simulink model "STEVE_ver28"  (R2022a)
settings: Solver=VariableStepAuto  StartTime=0.0  StopTime=Stop_Time  FixedStep=0.000001  RelTol=1e-5
values from neighbouring files (symbols this model uses):
  Bed_ave_OD = (1+Bed_ins_OD)/2    (= 1.667)    [STEVE_initialization.m]    (also in STEVE_running.m = (1+Bed_ins_OD)/2; STEVE_v4_C1Demo_2023_Nominal.m)
  Bed_ins_OD = 2.334    [STEVE_initialization.m]    (also in STEVE_v4_C1Demo_2023_Nominal.m)
  Bed_thickness = 0.049    [STEVE_initialization.m]    (also in STEVE_v4_C1Demo_2023_Nominal.m)
  Belimo_Cv = 16    [STEVE_initialization.m]    (also in STEVE_v4_C1Demo_2023_Nominal.m)
  flow_rate = 8    [STEVE_initialization.m]    (also in STEVE_v4_C1Demo_2023_Nominal.m)
  Heat_ads = 40000    [STEVE_initialization.m]    (also in STEVE_v4_C1Demo_2023_Nominal.m)
  Heater_output = 85.3    [STEVE_initialization.m]    (also in STEVE_v4_C1Demo_2023_Nominal.m)
  L = 0.508    [STEVE_initialization.m]    (also in STEVE_v4_C1Demo_2023_Nominal.m)
  L_inch = L*39.3701    (= 20.0000108)    [STEVE_initialization.m]    (also in STEVE_v4_C1Demo_2023_Nominal.m)
  max_temp = 200+273.15    (= 473.15)    [STEVE_initialization.m]    (also in STEVE_v4_C1Demo_2023_Nominal.m)
  mesh_size = 15    [STEVE_initialization.m]    (also in STEVE_v4_C1Demo_2023_Nominal.m)
  Pipe_ave_HD = (pipe_HD+0.5)/2    (= 0.465)    [STEVE_initialization.m]    (also in STEVE_running.m = (pipe_HD+0.5)/2; STEVE_v4_C1Demo_2023_Nominal.m)
  pipe_HD = 0.43    [STEVE_initialization.m]    (also in STEVE_v4_C1Demo_2023_Nominal.m)
  Ramp_rate = 0.0833    [STEVE_initialization.m]    (also in STEVE_v4_C1Demo_2023_Nominal.m)
  room_pressure = 13.3    [STEVE_initialization.m]    (also in STEVE_v4_C1Demo_2023_Nominal.m)
  t_Total = Adsorption_time + FlowStop_time + Valve_close_Time + Select_valve_close_Time + Pump_down_time + Desorption_time + SelectValve_open_Time + Valve_open_Time    (= 9635)    [STEVE_initialization.m]    (also in STEVE_running.m = Adsorption_time + FlowStop_time + Valve_close_Time + Select_; STEVE_v4_C1Demo_2023_Nominal.m)
libraries: fl_lib x229, nesl_utility x75, slpidlib x2
(part 5 of 5)

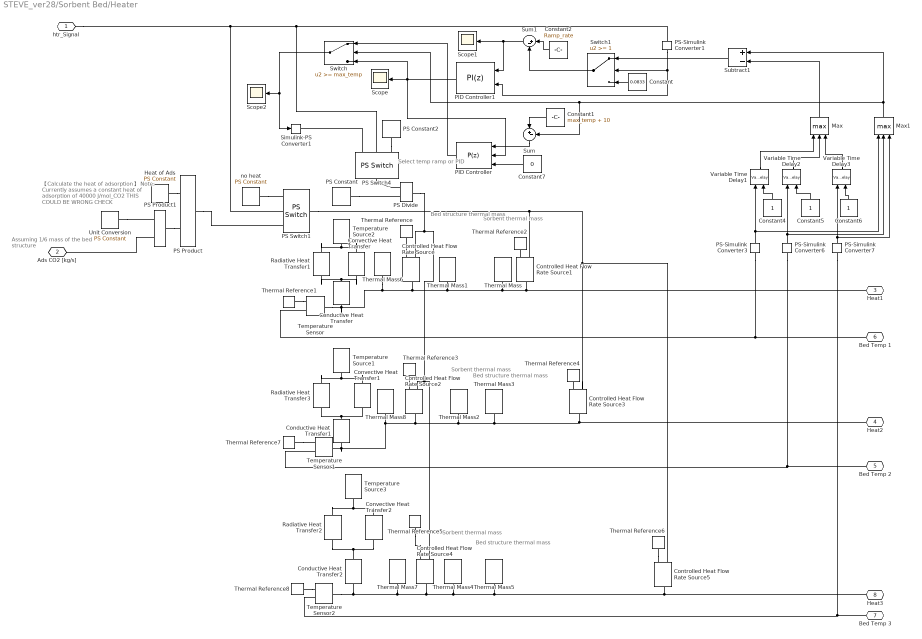
== system STEVE_ver28/Sorbent Bed/Heater ==
  note: 【Calculate the heat of adsorption】
      | Note: Currently assumes a constant heat of adsorption of 40000 J/mol_CO2
      | THIS COULD BE WRONG CHECK
  note: Sorbent thermal mass
  note: Bed structure thermal mass
  note: Bed structure thermal mass
  note: Sorbent thermal mass
  note: Bed structure thermal mass
  note: Sorbent thermal mass
  note: Select temp ramp or PID
  note: Assuming 1/6 mass of the bed structure
  Conductive Heat Transfer : fl_lib/Thermal/Thermal Elements/Conductive Heat Transfer  area=pi*Bed_ave_OD*L_inch/3 in^2  thickness=0.667 in  th_cond=0.07 W/(K*m)  T_specify=off  T_priority=None  T=0 K  T_nominal_specify=off  T_nominal_unit=K  T_nominal_value=1  Q_specify=off  Q_priority=None  Q=0 W  Q_nominal_specify=off  Q_nominal_unit=W  Q_nominal_value=1
      settings: SourceProductBaseCode=PW,SS,VE
  Conductive Heat Transfer1 : fl_lib/Thermal/Thermal Elements/Conductive Heat Transfer  area=pi*Bed_ave_OD*L_inch/3 in^2  thickness=0.667 in  th_cond=0.07 W/(K*m)  T_specify=off  T_priority=None  T=0 K  T_nominal_specify=off  T_nominal_unit=K  T_nominal_value=1  Q_specify=off  Q_priority=None  Q=0 W  Q_nominal_specify=off  Q_nominal_unit=W  Q_nominal_value=1
      settings: SourceProductBaseCode=PW,SS,VE
  Conductive Heat Transfer2 : fl_lib/Thermal/Thermal Elements/Conductive Heat Transfer  area=pi*Bed_ave_OD*L_inch/3 in^2  thickness=0.667 in  th_cond=0.07 W/(K*m)  T_specify=off  T_priority=None  T=0 K  T_nominal_specify=off  T_nominal_unit=K  T_nominal_value=1  Q_specify=off  Q_priority=None  Q=0 W  Q_nominal_specify=off  Q_nominal_unit=W  Q_nominal_value=1
      settings: SourceProductBaseCode=PW,SS,VE
  Constant : Constant  Value=0.0833
  Constant1 : Constant  Value=max_temp + 10
  Constant2 : Constant  Value=Ramp_rate
  Constant4 : Constant
  Constant5 : Constant
  Constant6 : Constant
  Constant7 : Constant  Value=0
  Controlled Heat Flow Rate Source{,1..5} (6 alike) : fl_lib/Thermal/Thermal Sources/Controlled Heat Flow Rate Source
      settings: SourceProductBaseCode=PW,SS,VE
  Convective Heat Transfer : fl_lib/Thermal/Thermal Elements/Convective Heat Transfer  area=pi*Bed_ins_OD*L_inch/3 in^2  heat_tr_coeff=5 W/(K*m^2)  T_specify=off  T_priority=None  T=0 K  T_nominal_specify=off  T_nominal_unit=K  T_nominal_value=1  Q_specify=off  Q_priority=None  Q=0 W  Q_nominal_specify=off  Q_nominal_unit=W  Q_nominal_value=1
      settings: SourceProductBaseCode=PW,SS,VE
  Convective Heat Transfer1 : fl_lib/Thermal/Thermal Elements/Convective Heat Transfer  area=pi*Bed_ins_OD*L_inch/3 in^2  heat_tr_coeff=5 W/(K*m^2)  T_specify=off  T_priority=None  T=0 K  T_nominal_specify=off  T_nominal_unit=K  T_nominal_value=1  Q_specify=off  Q_priority=None  Q=0 W  Q_nominal_specify=off  Q_nominal_unit=W  Q_nominal_value=1
      settings: SourceProductBaseCode=PW,SS,VE
  Convective Heat Transfer2 : fl_lib/Thermal/Thermal Elements/Convective Heat Transfer  area=pi*Bed_ins_OD*L_inch/3 in^2  heat_tr_coeff=5 W/(K*m^2)  T_specify=off  T_priority=None  T=0 K  T_nominal_specify=off  T_nominal_unit=K  T_nominal_value=1  Q_specify=off  Q_priority=None  Q=0 W  Q_nominal_specify=off  Q_nominal_unit=W  Q_nominal_value=1
      settings: SourceProductBaseCode=PW,SS,VE
  Heat of Ads : fl_lib/Physical Signals/Sources/PS Constant  constant=Heat_ads/3 J/mol
      settings: SourceProductBaseCode=PW,SS,VE
  Max : MinMax  Function=max  Inputs=3
  Max1 : MinMax  Function=max  Inputs=3
  PID Controller : slpidlib/PID Controller  Controller=P  Form=Parallel  TimeDomain=Discrete-time  UseExternalTs=off  SampleTime=-1  IntegratorMethod=Forward Euler  FilterMethod=Forward Euler  ControllerParametersSource=internal  P=20  I=1  UseKiTs=on  D=0  N=100  UseFilter=on  TunerSelectOption=Transfer Function Based (PID Tuner App)  InitialConditionSource=internal  InitialConditionForIntegrator=0  InitialConditionForFilter=0  DifferentiatorICPrevScaledInput=0  ExternalReset=rising  TrackingMode=off  Kt=1  LimitOutput=on  SatLimitsSource=external  UpperSaturationLimit=60  LowerSaturationLimit=0  LinearizeAsGain=on  AntiWindupMode=none  Kb=1  POutMin=[]  POutMax=[]  IOutMin=[]  IOutMax=[]  DOutMin=[]  DOutMax=[]  NOutMin=[]  NOutMax=[]  SumOutMin=[]  SumOutMax=[]  SaturationOutMin=[]  SaturationOutMax=[]  PParamMin=[]  PParamMax=[]  IParamMin=[]  IParamMax=[]  DParamMin=[]  DParamMax=[]  NParamMin=[]  NParamMax=[]  KbParamMin=[]  KbParamMax=[]  KtParamMin=[]  KtParamMax=[]  KbOutMin=[]  KbOutMax=[]  KtOutMin=[]  KtOutMax=[]  IntegratorOutMin=[]  IntegratorOutMax=[]  FilterOutMin=[]  FilterOutMax=[]  SumI1OutMin=[]  SumI1OutMax=[]  SumI2OutMin=[]  SumI2OutMax=[]  SumI3OutMin=[]  SumI3OutMax=[]  SumI4OutMin=[]  SumI4OutMax=[]  SumDOutMin=[]  SumDOutMax=[]  DifferentiatorOutMin=[]  DifferentiatorOutMax=[]  FilterDiffOutCoefMin=[]  FilterDiffOutCoefMax=[]  ReciprocalOutMin=[]  ReciprocalOutMax=[]  SumDenOutMin=[]  SumDenOutMax=[]  SumNumOutMin=[]  SumNumOutMax=[]  DivideOutMin=[]  DivideOutMax=[]  UdiffTsProdOutMin=[]  UdiffTsProdOutMax=[]  NTsProdOutMin=[]  NTsProdOutMax=[]  UintegralTsProdOutMin=[]  UintegralTsProdOutMax=[]  UngainTsProdOutMin=[]  UngainTsProdOutMax=[]  ClampingZeroOutDataTypeStr=Inherit: Inherit via back propagation  ClampingZeroOutMin=[]  ClampingZeroOutMax=[]  FilterDenConstantOutDataTypeStr=Inherit: Inherit via back propagation  FilterDenConstantOutMin=[]  FilterDenConstantOutMax=[]  PCopyOutDataTypeStr=Inherit: Inherit via back propagation  PCopyOutMin=[]  PCopyOutMax=[]  NCopyOutDataTypeStr=Inherit: Inherit via back propagation  NCopyOutMin=[]  NCopyOutMax=[]  IntegratorContinuousStateAttributes=''  IntegratorStateMustResolveToSignalObject=off  IntegratorRTWStateStorageClass=Auto  FilterContinuousStateAttributes=''  FilterStateMustResolveToSignalObject=off  FilterRTWStateStorageClass=Auto  ParallelPVariant=InternalParameters  IdealPVariant=Disabled  IVariant=Disabled  DVariant=Disabled  IntegratorVariant=Disabled  SatVariant=External  AWVariant=Disabled  PCopyVariant=Disabled  TRVariant=Disabled  FdbkBlocksVariant=Forward  IdealPFdbkVariant=Disabled  SatFdbkVariant=Disabled  DerivativeFilterVariant=Disabled  NVariant=Disabled  NCopyVariant=Disabled_SignalSpec  FilterICVariant=Disabled  IntegratorICVariant=Disabled  ExternalResetVariant=Disabled  TRSumVariant=Passthrough  SumFdbkVariant=Disabled  SumVariant=Passthrough_P  TsampFilterVariant=InternalTs  TsampNgainVariant=Passthrough  TsampIntegralVariant=Disabled_SignalSpec  ExternalSaturationOutDataTypeStr=Inherit: Same as second input  aMode=0
  PID Controller1 : slpidlib/PID Controller  Controller=PI  Form=Parallel  TimeDomain=Discrete-time  UseExternalTs=off  SampleTime=-1  IntegratorMethod=Forward Euler  FilterMethod=Forward Euler  ControllerParametersSource=internal  P=500  I=50  UseKiTs=on  D=0  N=100  UseFilter=on  TunerSelectOption=Transfer Function Based (PID Tuner App)  InitialConditionSource=internal  InitialConditionForIntegrator=0  InitialConditionForFilter=0  DifferentiatorICPrevScaledInput=0  ExternalReset=either  TrackingMode=off  Kt=1  LimitOutput=on  SatLimitsSource=internal  UpperSaturationLimit=Heater_output  LowerSaturationLimit=0  LinearizeAsGain=on  AntiWindupMode=none  Kb=1  POutMin=[]  POutMax=[]  IOutMin=[]  IOutMax=[]  DOutMin=[]  DOutMax=[]  NOutMin=[]  NOutMax=[]  SumOutMin=[]  SumOutMax=[]  SaturationOutMin=[]  SaturationOutMax=[]  PParamMin=[]  PParamMax=[]  IParamMin=[]  IParamMax=[]  DParamMin=[]  DParamMax=[]  NParamMin=[]  NParamMax=[]  KbParamMin=[]  KbParamMax=[]  KtParamMin=[]  KtParamMax=[]  KbOutMin=[]  KbOutMax=[]  KtOutMin=[]  KtOutMax=[]  IntegratorOutMin=[]  IntegratorOutMax=[]  FilterOutMin=[]  FilterOutMax=[]  SumI1OutMin=[]  SumI1OutMax=[]  SumI2OutMin=[]  SumI2OutMax=[]  SumI3OutMin=[]  SumI3OutMax=[]  SumI4OutMin=[]  SumI4OutMax=[]  SumDOutMin=[]  SumDOutMax=[]  DifferentiatorOutMin=[]  DifferentiatorOutMax=[]  FilterDiffOutCoefMin=[]  FilterDiffOutCoefMax=[]  ReciprocalOutMin=[]  ReciprocalOutMax=[]  SumDenOutMin=[]  SumDenOutMax=[]  SumNumOutMin=[]  SumNumOutMax=[]  DivideOutMin=[]  DivideOutMax=[]  UdiffTsProdOutMin=[]  UdiffTsProdOutMax=[]  NTsProdOutMin=[]  NTsProdOutMax=[]  UintegralTsProdOutMin=[]  UintegralTsProdOutMax=[]  UngainTsProdOutMin=[]  UngainTsProdOutMax=[]  ClampingZeroOutDataTypeStr=Inherit: Inherit via back propagation  ClampingZeroOutMin=[]  ClampingZeroOutMax=[]  FilterDenConstantOutDataTypeStr=Inherit: Inherit via back propagation  FilterDenConstantOutMin=[]  FilterDenConstantOutMax=[]  PCopyOutDataTypeStr=Inherit: Inherit via back propagation  PCopyOutMin=[]  PCopyOutMax=[]  NCopyOutDataTypeStr=Inherit: Inherit via back propagation  NCopyOutMin=[]  NCopyOutMax=[]  IntegratorContinuousStateAttributes=''  IntegratorStateMustResolveToSignalObject=off  IntegratorRTWStateStorageClass=Auto  FilterContinuousStateAttributes=''  FilterStateMustResolveToSignalObject=off  FilterRTWStateStorageClass=Auto  ParallelPVariant=InternalParameters  IdealPVariant=Disabled  IVariant=InternalParameters  DVariant=Disabled  IntegratorVariant=Discrete  SatVariant=Enabled  AWVariant=Passthrough  PCopyVariant=Disabled  TRVariant=Disabled  FdbkBlocksVariant=Forward  IdealPFdbkVariant=Disabled  SatFdbkVariant=Disabled  DerivativeFilterVariant=Disabled  NVariant=Disabled  NCopyVariant=Disabled_SignalSpec  FilterICVariant=Disabled  IntegratorICVariant=InternalICs  ExternalResetVariant=ExternalReset  TRSumVariant=Passthrough  SumFdbkVariant=Disabled  SumVariant=Sum_PI  TsampFilterVariant=InternalTs  TsampNgainVariant=Passthrough  TsampIntegralVariant=Passthrough  ExternalSaturationOutDataTypeStr=Inherit: Same as second input  aMode=0
  PS Constant : fl_lib/Physical Signals/Sources/PS Constant  constant=3
      settings: SourceProductBaseCode=PW,SS,VE
  PS Constant2 : fl_lib/Physical Signals/Sources/PS Constant  constant=0
      settings: SourceProductBaseCode=PW,SS,VE
  PS Divide : fl_lib/Physical Signals/Functions/PS Divide
      settings: SourceProductBaseCode=PW,SS,VE
  PS Product : fl_lib/Physical Signals/Functions/PS Product
      settings: SourceProductBaseCode=PW,SS,VE
  PS Product1 : fl_lib/Physical Signals/Functions/PS Product
      settings: SourceProductBaseCode=PW,SS,VE
  PS Switch1 : fl_lib/Physical Signals/Nonlinear Operators/PS Switch  Threshold=1
      settings: SourceProductBaseCode=PW,SS,VE  InternalSimscapePortConfiguration="{\"Bottom\":[],\"Left\":[{\"id\":\"I1\",\"label\":\"\",\"type\":\"input\"},{\"id\":\"I2\",\"label\":\"\",\"type\":\"input\"},{\"id\":\"I3\",\"label\":\"\",\"type\":\"input\"}],\"Right\":[{\"id\":\"O\",\"label\":\"\",\"type\":\"output\"}],\"Top\":[]}"
  PS Switch4 : fl_lib/Physical Signals/Nonlinear Operators/PS Switch  Threshold=1
      settings: SourceProductBaseCode=PW,SS,VE  InternalSimscapePortConfiguration="{\"Bottom\":[],\"Left\":[{\"id\":\"I1\",\"label\":\"\",\"type\":\"input\"},{\"id\":\"I2\",\"label\":\"\",\"type\":\"input\"},{\"id\":\"I3\",\"label\":\"\",\"type\":\"input\"}],\"Right\":[{\"id\":\"O\",\"label\":\"\",\"type\":\"output\"}],\"Top\":[]}"
  PS-Simulink Converter{1,3,6..7} (4 alike) : nesl_utility/PS-Simulink Converter  PhysicalDomain=network_engine_domain  SubClassName=ps_output  LeftPortType=input  RightPortType=output  PseudoPeriodic=off  Frequencies=[]  VectorFormat=inherit  Unit=K  AffineConversion=off
      settings: SourceProductBaseCode=SS,PW,VE
  Radiative Heat Transfer1 : fl_lib/Thermal/Thermal Elements/Radiative Heat Transfer  area=pi*Bed_ins_OD*L_inch/3 in^2  rad_tr_coeff=5.67e-8 W/(K^4*m^2)  T_specify=off  T_priority=None  T=0 K  T_nominal_specify=off  T_nominal_unit=K  T_nominal_value=1  Q_specify=off  Q_priority=None  Q=0 W  Q_nominal_specify=off  Q_nominal_unit=W  Q_nominal_value=1
      settings: SourceProductBaseCode=PW,SS,VE  InternalSimscapePortConfiguration="{\"Bottom\":[],\"Left\":[{\"id\":\"A\",\"label\":\"A\",\"type\":\"foundation.thermal.thermal\"}],\"Right\":[{\"id\":\"B\",\"label\":\"B\",\"type\":\"foundation.thermal.thermal\"}],\"Top\":[]}"
  Radiative Heat Transfer2 : fl_lib/Thermal/Thermal Elements/Radiative Heat Transfer  area=pi*Bed_ins_OD*L_inch/3 in^2  rad_tr_coeff=5.67e-8 W/(K^4*m^2)  T_specify=off  T_priority=None  T=0 K  T_nominal_specify=off  T_nominal_unit=K  T_nominal_value=1  Q_specify=off  Q_priority=None  Q=0 W  Q_nominal_specify=off  Q_nominal_unit=W  Q_nominal_value=1
      settings: SourceProductBaseCode=PW,SS,VE  InternalSimscapePortConfiguration="{\"Bottom\":[],\"Left\":[{\"id\":\"A\",\"label\":\"A\",\"type\":\"foundation.thermal.thermal\"}],\"Right\":[{\"id\":\"B\",\"label\":\"B\",\"type\":\"foundation.thermal.thermal\"}],\"Top\":[]}"
  Radiative Heat Transfer3 : fl_lib/Thermal/Thermal Elements/Radiative Heat Transfer  area=pi*Bed_ins_OD*L_inch/3 in^2  rad_tr_coeff=5.67e-8 W/(K^4*m^2)  T_specify=off  T_priority=None  T=0 K  T_nominal_specify=off  T_nominal_unit=K  T_nominal_value=1  Q_specify=off  Q_priority=None  Q=0 W  Q_nominal_specify=off  Q_nominal_unit=W  Q_nominal_value=1
      settings: SourceProductBaseCode=PW,SS,VE  InternalSimscapePortConfiguration="{\"Bottom\":[],\"Left\":[{\"id\":\"A\",\"label\":\"A\",\"type\":\"foundation.thermal.thermal\"}],\"Right\":[{\"id\":\"B\",\"label\":\"B\",\"type\":\"foundation.thermal.thermal\"}],\"Top\":[]}"
  Scope : Scope
  Scope1 : Scope
  Scope2 : Scope
  Simulink-PS Converter1 : nesl_utility/Simulink-PS Converter  PhysicalDomain=network_engine_domain  SubClassName=ps_input  LeftPortType=input  RightPortType=output  PseudoPeriodic=off  Frequencies=[]  NoiseDistribution=none  NoiseParameters=[]  Unit=1  AffineConversion=off  FilteringAndDerivatives=provide  SimscapeFilterOrder=1  InputFilterTimeConstant=0.001  UdotUserProvided=0
      settings: SourceProductBaseCode=SS,PW,VE
  Subtract1 : Sum  Inputs=+-
  Sum : Sum  Inputs=|+-
  Sum1 : Sum  Inputs=|+-
  Switch : Switch  Threshold=max_temp  SaturateOnIntegerOverflow=off  InputSameDT=off
  Switch1 : Switch  Threshold=1  SaturateOnIntegerOverflow=off  InputSameDT=off
  Temperature Sensor : fl_lib/Thermal/Thermal Sensors/Temperature Sensor
      settings: SourceProductBaseCode=PW,SS,VE
  Temperature Sensor1 : fl_lib/Thermal/Thermal Sensors/Temperature Sensor
      settings: SourceProductBaseCode=PW,SS,VE
  Temperature Sensor2 : fl_lib/Thermal/Thermal Sensors/Temperature Sensor
      settings: SourceProductBaseCode=PW,SS,VE
  Temperature Source1 : fl_lib/Thermal/Thermal Sources/Temperature Source  temperature=room_temp K
      settings: SourceProductBaseCode=PW,SS,VE
  Temperature Source2 : fl_lib/Thermal/Thermal Sources/Temperature Source  temperature=room_temp K
      settings: SourceProductBaseCode=PW,SS,VE
  Temperature Source3 : fl_lib/Thermal/Thermal Sources/Temperature Source  temperature=room_temp K
      settings: SourceProductBaseCode=PW,SS,VE
  Thermal Mass : fl_lib/Thermal/Thermal Elements/Thermal Mass  mass=110.5/3 g  sp_heat=500 J/kg/K  T_specify=off  T_priority=High  T=300 K  T_nominal_specify=off  T_nominal_unit=K  T_nominal_value=1  Q_specify=off  Q_priority=None  Q=0 W  Q_nominal_specify=off  Q_nominal_unit=W  Q_nominal_value=1
      settings: SourceProductBaseCode=PW,SS,VE
  Thermal Mass1 : fl_lib/Thermal/Thermal Elements/Thermal Mass  mass=313/3 g  sp_heat=490 J/kg/K  T_specify=off  T_priority=High  T=300 K  T_nominal_specify=off  T_nominal_unit=K  T_nominal_value=1  Q_specify=off  Q_priority=None  Q=0 W  Q_nominal_specify=off  Q_nominal_unit=W  Q_nominal_value=1
      settings: SourceProductBaseCode=PW,SS,VE
  Thermal Mass2 : fl_lib/Thermal/Thermal Elements/Thermal Mass  mass=110.5/3 g  sp_heat=500 J/kg/K  T_specify=off  T_priority=High  T=300 K  T_nominal_specify=off  T_nominal_unit=K  T_nominal_value=1  Q_specify=off  Q_priority=None  Q=0 W  Q_nominal_specify=off  Q_nominal_unit=W  Q_nominal_value=1
      settings: SourceProductBaseCode=PW,SS,VE
  Thermal Mass3 : fl_lib/Thermal/Thermal Elements/Thermal Mass  mass=313/3 g  sp_heat=490 J/kg/K  T_specify=off  T_priority=High  T=300 K  T_nominal_specify=off  T_nominal_unit=K  T_nominal_value=1  Q_specify=off  Q_priority=None  Q=0 W  Q_nominal_specify=off  Q_nominal_unit=W  Q_nominal_value=1
      settings: SourceProductBaseCode=PW,SS,VE
  Thermal Mass4 : fl_lib/Thermal/Thermal Elements/Thermal Mass  mass=110.5/3 g  sp_heat=500 J/kg/K  T_specify=off  T_priority=High  T=300 K  T_nominal_specify=off  T_nominal_unit=K  T_nominal_value=1  Q_specify=off  Q_priority=None  Q=0 W  Q_nominal_specify=off  Q_nominal_unit=W  Q_nominal_value=1
      settings: SourceProductBaseCode=PW,SS,VE
  Thermal Mass5 : fl_lib/Thermal/Thermal Elements/Thermal Mass  mass=313/3 g  sp_heat=490 J/kg/K  T_specify=off  T_priority=High  T=300 K  T_nominal_specify=off  T_nominal_unit=K  T_nominal_value=1  Q_specify=off  Q_priority=None  Q=0 W  Q_nominal_specify=off  Q_nominal_unit=W  Q_nominal_value=1
      settings: SourceProductBaseCode=PW,SS,VE
  Thermal Mass6 : fl_lib/Thermal/Thermal Elements/Thermal Mass  mass=313/6 g  sp_heat=960 J/kg/K  T_specify=off  T_priority=High  T=300 K  T_nominal_specify=off  T_nominal_unit=K  T_nominal_value=1  Q_specify=off  Q_priority=None  Q=0 W  Q_nominal_specify=off  Q_nominal_unit=W  Q_nominal_value=1
      settings: SourceProductBaseCode=PW,SS,VE
  Thermal Mass7 : fl_lib/Thermal/Thermal Elements/Thermal Mass  mass=313/6 g  sp_heat=960 J/kg/K  T_specify=off  T_priority=High  T=300 K  T_nominal_specify=off  T_nominal_unit=K  T_nominal_value=1  Q_specify=off  Q_priority=None  Q=0 W  Q_nominal_specify=off  Q_nominal_unit=W  Q_nominal_value=1
      settings: SourceProductBaseCode=PW,SS,VE
  Thermal Mass8 : fl_lib/Thermal/Thermal Elements/Thermal Mass  mass=313/6 g  sp_heat=960 J/kg/K  T_specify=off  T_priority=High  T=300 K  T_nominal_specify=off  T_nominal_unit=K  T_nominal_value=1  Q_specify=off  Q_priority=None  Q=0 W  Q_nominal_specify=off  Q_nominal_unit=W  Q_nominal_value=1
      settings: SourceProductBaseCode=PW,SS,VE
  Thermal Reference{,1..8} (9 alike) : fl_lib/Thermal/Thermal Elements/Thermal Reference
      settings: SourceProductBaseCode=PW,SS,VE
  Unit Conversion : fl_lib/Physical Signals/Sources/PS Constant  constant=-1000/44 mol/kg
      settings: SourceProductBaseCode=PW,SS,VE
  Variable Time Delay1 : VariableTransportDelay  MaximumDelay=10
  Variable Time Delay2 : VariableTransportDelay  MaximumDelay=10
  Variable Time Delay3 : VariableTransportDelay  MaximumDelay=10
  no heat : fl_lib/Physical Signals/Sources/PS Constant  constant=0 J/s
      settings: SourceProductBaseCode=PW,SS,VE
  htr_Signal : PMIOPort  Side=Left
  Ads CO2 [kg/s] : PMIOPort  Port=2  Side=Left
  Heat1 : PMIOPort  Port=3  Side=Left
  Heat2 : PMIOPort  Port=4  Side=Left
  Bed Temp 2 : PMIOPort  Port=5  Side=Right
  Bed Temp 1 : PMIOPort  Port=6  Side=Right
  Bed Temp 3 : PMIOPort  Port=7  Side=Right
  Heat3 : PMIOPort  Port=8  Side=Right
  wires:
  PID Controller1/1 -> PID Controller/2, Scope/1, Switch/3
  Constant1/1 -> Sum/1
  Sum1/1 -> PID Controller1/1, Scope1/1
  Sum/1 -> PID Controller/1
  PID Controller/1 -> Switch/1
  Max1/1 -> Sum/2, Switch/2, Subtract1/1
  Constant2/1 -> Sum1/1
  Constant/1 -> Switch1/3
  PS-Simulink Converter1/1 -> Switch1/2, PID Controller1/2
  Constant4/1 -> Variable Time Delay1/2
  PS-Simulink Converter3/1 -> Variable Time Delay1/1, Max1/1
  Constant5/1 -> Variable Time Delay2/2
  PS-Simulink Converter6/1 -> Variable Time Delay2/1, Max1/2
  Constant6/1 -> Variable Time Delay3/2
  PS-Simulink Converter7/1 -> Max1/3, Variable Time Delay3/1
  Variable Time Delay1/1 -> Max/1
  Variable Time Delay2/1 -> Max/2
  Variable Time Delay3/1 -> Max/3
  Max/1 -> Subtract1/2
  Subtract1/1 -> Switch1/1
  Switch1/1 -> Sum1/2
  Constant7/1 -> PID Controller/3
  Switch/1 -> Scope2/1, Simulink-PS Converter1/1
  connections:
  PS Product1/RConn1 -- PS Product/LConn2
  Unit Conversion/RConn1 -- PS Product1/LConn1
  PS Product1/LConn2 -- Ads CO2 [kg/s]/RConn1
  Heat of Ads/RConn1 -- PS Product/LConn1
  Thermal Reference/LConn1 -- Controlled Heat Flow Rate Source/RConn2
  Thermal Reference1/LConn1 -- Temperature Sensor/RConn1
  Controlled Heat Flow Rate Source/LConn1 -- Thermal Mass1/LConn1 -- Thermal Mass/LConn1 -- Controlled Heat Flow Rate Source1/LConn1 -- Heat1/RConn1 -- Temperature Sensor/LConn1 -- Conductive Heat Transfer/LConn1 -- Thermal Mass6/LConn1
  Thermal Reference2/LConn1 -- Controlled Heat Flow Rate Source1/RConn2
  PS-Simulink Converter3/LConn1 -- Bed Temp 1/RConn1 -- Temperature Sensor/RConn2
  Thermal Reference7/LConn1 -- Temperature Sensor1/RConn1
  Thermal Reference8/LConn1 -- Temperature Sensor2/RConn1
  Temperature Sensor1/RConn2 -- PS-Simulink Converter6/LConn1 -- Bed Temp 2/RConn1
  Bed Temp 3/RConn1 -- PS-Simulink Converter7/LConn1 -- Temperature Sensor2/RConn2
  Thermal Mass2/LConn1 -- Controlled Heat Flow Rate Source3/LConn1 -- Heat2/RConn1 -- Thermal Mass3/LConn1 -- Conductive Heat Transfer1/LConn1 -- Temperature Sensor1/LConn1 -- Thermal Mass8/LConn1 -- Controlled Heat Flow Rate Source2/LConn1
  Thermal Reference3/LConn1 -- Controlled Heat Flow Rate Source2/RConn2
  Thermal Reference4/LConn1 -- Controlled Heat Flow Rate Source3/RConn2
  Temperature Sensor2/LConn1 -- Heat3/RConn1 -- Controlled Heat Flow Rate Source5/LConn1 -- Thermal Mass5/LConn1 -- Thermal Mass4/LConn1 -- Controlled Heat Flow Rate Source4/LConn1 -- Thermal Mass7/LConn1 -- Conductive Heat Transfer2/LConn1
  Thermal Reference6/LConn1 -- Controlled Heat Flow Rate Source5/RConn2
  Thermal Reference5/LConn1 -- Controlled Heat Flow Rate Source4/RConn2
  htr_Signal/RConn1 -- PS-Simulink Converter1/LConn1 -- PS Switch4/LConn2 -- PS Switch1/LConn2
  PS Switch4/LConn1 -- Simulink-PS Converter1/RConn1
  PS Constant2/RConn1 -- PS Switch4/LConn3
  Controlled Heat Flow Rate Source3/RConn1 -- Controlled Heat Flow Rate Source5/RConn1 -- PS Switch1/RConn1 -- Controlled Heat Flow Rate Source1/RConn1
  no heat/RConn1 -- PS Switch1/LConn1
  Convective Heat Transfer/LConn1 -- Radiative Heat Transfer1/LConn1 -- Conductive Heat Transfer/RConn1
  Convective Heat Transfer/RConn1 -- Radiative Heat Transfer1/RConn1 -- Temperature Source2/LConn1
  Convective Heat Transfer1/LConn1 -- Radiative Heat Transfer3/LConn1 -- Conductive Heat Transfer1/RConn1
  Convective Heat Transfer1/RConn1 -- Radiative Heat Transfer3/RConn1 -- Temperature Source1/LConn1
  Convective Heat Transfer2/LConn1 -- Conductive Heat Transfer2/RConn1 -- Radiative Heat Transfer2/LConn1
  Radiative Heat Transfer2/RConn1 -- Temperature Source3/LConn1 -- Convective Heat Transfer2/RConn1
  PS Product/RConn1 -- PS Switch1/LConn3
  PS Divide/RConn1 -- Controlled Heat Flow Rate Source/RConn1 -- Controlled Heat Flow Rate Source2/RConn1 -- Controlled Heat Flow Rate Source4/RConn1
  PS Divide/LConn1 -- PS Switch4/RConn1
  PS Constant/RConn1 -- PS Divide/LConn2

== system STEVE_ver28/Subsystem1/Pump Exhaust ==
  note: Only send in CO2 during desorption
  PS Constant2 : fl_lib/Physical Signals/Sources/PS Constant  constant=0 kg/s
      settings: SourceProductBaseCode=PW,SS,VE
  PS Switch : fl_lib/Physical Signals/Nonlinear Operators/PS Switch  Threshold=1
      settings: SourceProductBaseCode=PW,SS,VE  InternalSimscapePortConfiguration="{\"Bottom\":[],\"Left\":[{\"id\":\"I1\",\"label\":\"\",\"type\":\"input\"},{\"id\":\"I2\",\"label\":\"\",\"type\":\"input\"},{\"id\":\"I3\",\"label\":\"\",\"type\":\"input\"}],\"Right\":[{\"id\":\"O\",\"label\":\"\",\"type\":\"output\"}],\"Top\":[]}"
  Des CO2 out : PMIOPort  Side=Left
  Signal : PMIOPort  Port=2  Side=Left
  signal1 : PMIOPort  Port=3  Side=Right
  connections:
  Des CO2 out/RConn1 -- PS Switch/LConn1
  PS Switch/LConn2 -- Signal/RConn1
  PS Constant2/RConn1 -- PS Switch/LConn3
  PS Switch/RConn1 -- signal1/RConn1

== matlab function STEVE_ver28/Subsystem/Valve 204 ==
  data: V input; M input; sig input; P input; T input; valve_o_c input; D input; A output; dP output; Cv input; t input
function [A,dP] = fcn( V, M, sig, P, T, valve_o_c, D, Cv, t)


%calculate local resctriction area
 
if valve_o_c==0 
    
    A=1e-10;
    dP=0;
else


if t<1
    A=((pi*(D-0.0001)^2)/4);
    dP=0;
else
    %A=((pi*(D-0.0001)^2)/4)*(valve_o_c/90);
    A=((pi*(D-0.0001)^2)/4)*((1e-3)*(valve_o_c/18)/90);
    dP=0;
end

end







%         if valve_o_c<=8
%             A=1e-10; 
%             roh_air=1.225; % Air density [kg/m^3]
%             G=(M/V)/roh_air; %Specific gravity. (Volumetric Flow Rate)/(Mass Flow Rate)
%             Cv=0.0001;%Prevents flow. Cannot set Cv to zero because it violates the assumption of conservation of mass
%             Q=V/0.0000079; %Convert m^3/s to SCFH
%             TF=(T-273.15)*9/5+32;%Convert Kelvin into F
%           % u_psi=(P/6894.76)-sqrt((P/6894.76)^2-(G*(TF+460)*(Q/(963*Cv))^2));%Calculate pressure drop in [psi] (Ref:https://www.engvalves.com/core/medialibrary/engvalves/website/Tools-Resources/Brochures/DiaFlo/DVComputations.pdf?ext=.pdf)
%           % u=u_psi*6894.76; % Convert deltaP unit from psi to [Pa]        
% 
%         elseif valve_o_c==90
%             valve_o_c=89.9999;
%             h=valve_o_c*r*2/90;
%             theta=2*acos(1-(h/r));
%             A=(theta/2)*(r^2)-(r-h)*sqrt(h*(2*r-h));
%             A_max=pi*r^2;
%             A_ratio=A/A_max;
%             Cv=Cv*A_ratio;
% 
%             roh_air=1.225; % Air density [kg/m^3]
%             G=(M/V)/roh_air; %Specific gravity. (Volumetric Flow Rate)/(Mass Flow Rate)
%             Q=V/0.0000079; %Convert m^3/s to SCFH
%             TF=(T-273.15)*9/5+32;%Convert Kelvin into F
%             % u_psi=(P/6894.76)-sqrt((P/6894.76)^2-(G*(TF+460)*(Q/(963*Cv))^2));%Calculate pressure drop in [psi] (Ref:https://www.engvalves.com/core/medialibrary/engvalves/website/Tools-Resources/Brochures/DiaFlo/DVComputations.pdf?ext=.pdf)
%            %  u=u_psi*6894.76; % Convert deltaP unit from psi to [Pa]
% 
%         else
%             h=(valve_o_c)*r*2/90;
%             theta=2*acos(1-(h/r));
%             A=(theta/2)*(r^2)-(r-h)*sqrt(h*(2*r-h));
%             A_max=pi*r^2;
%             A_ratio=A/A_max;
%             Cv=Cv*A_ratio;
% 
%             roh_air=1.225; % Air density [kg/m^3]
%             G=(M/V)/roh_air; %Specific gravity. (Volumetric Flow Rate)/(Mass Flow Rate)
%             Q=V/0.0000079; %Convert m^3/s to SCFH
%             TF=(T-273.15)*9/5+32;%Convert Kelvin into F
%           %   u_psi=(P/6894.76)-sqrt((P/6894.76)^2-(G*(TF+460)*(Q/(963*Cv))^2));%Calculate pressure drop in [psi] (Ref:https://www.engvalves.com/core/medialibrary/engvalves/website/Tools-Resources/Brochures/DiaFlo/DVComputations.pdf?ext=.pdf)
%           %   u=u_psi*6894.76; % Convert deltaP unit from psi to [Pa]
%             
%         end

%         if t<=1
%             dP=0;
%         else
%             if  V>0
%                 dP=-u; %Need a negative to simulate pressure drop from the port A to B direction
%             else
%                 dP=0;
%             end
%         end


%Other parameter units
%V: Flow Rate [m^3/s]
%P: Pressure [Pa]
%x: Valve initial position [deg]
%x_fin: Final Valve position [deg]
%t_dur: Time it takes to the valve to rotate to teh commanded position [s]
%t_start: Time to start changing valve position [s]
%t: Simulation time [s]
%M: Mixture mass flow rate [kg/s]
%x_fin: Valve final position [deg]
%T:Temperature [K]

== matlab function STEVE_ver28/DAQ/Downstream Flow Rate ==
  settings: updateMethod=DISCRETE  sampleTime=1
  data: FMdown output; x input; s input
function FMdown  = fcn(x,s)
%rng shuffle
range=10;
sigma=0.002*range+0.008*abs(x);

FM=normrnd(x,sigma/3,[1,1000]);
FMdown=FM(1,s);

== matlab function STEVE_ver28/DAQ/Filter Pressure Drop ==
  settings: updateMethod=DISCRETE  sampleTime=1
  data: dP output; x input
function dP  = fcn(x)
%rng shuffle

x=x/6894; %Pa to psi
sigma=0.0008*abs(x);
dP_pre=normrnd(x,sigma/3,[1,5]);
dP=dP_pre(5);

== matlab function STEVE_ver28/Filter/Check Valve ==
  data: V input; reg output; P input; dP output
function [reg,dP] = fcn(V,P)


%Check valve closed
if P<=2275.27 %Pa
    reg=1^(-10)*39.3701; % Unit conversion. m to in
    dP=0; % Not sure if this is accurate. Probably doesn't matter though
%Check valve open
else
V=V*246.172; % m^3 to gallon
Cv=1.68; %Specification -> https://www.mcmaster.com/45385K56/
G=1; %Specific gravity
dP=(V/Cv)^2*G; % DeltaP[Pa], V -> m^3/s   
reg=0.12799999; %in^2
dP=-dP % chage it to negative value so that it would cause pressure "drop"
end

== matlab function STEVE_ver28/Filter/Calculate pressure drop across a filter ==
  data: dP output; mesh input; sig input

function dP = fcn(mesh, sig)

%Caution: THIS IS EMPIRICAL!!!!!!
if sig==1
    dP=0;
else

    if mesh==60 %μm
        dP=-0.1*6894.76; % convert 0.1psi to Pa
    elseif mesh==15
        dP=-0.15*6894.76; % convert 0.1psi to Pa 
    elseif mesh==2
        dP=-0.2*6894.76;% convert 0.1psi to Pa 
    else %Custom
        dP=-1.8*6894.76;% convert 0.1psi to Pa 
    end
end

== matlab function STEVE_ver28/DAQ/Bed Pressure Drop ==
  settings: updateMethod=DISCRETE  sampleTime=1
  data: dP output; x input
function dP  = fcn(x)
%rng shuffle
x=x/6894; %Pa to psi

sigma=0.0008*abs(x);

dP_pre=normrnd(x,sigma/3,[1,6]);
dP=dP_pre(6);

== matlab function STEVE_ver28/Sorbent Bed/CO2 Desorption/Cycle Counter ==
  data: t input; t_tot input; in input; out output; time output
function [out,time]  = fcn(t,t_tot,in)

cycle=floor(t/t_tot);  
time= t-t_tot*cycle;
if time <=5
    out=0;
else
    out=in;
  
  end

== matlab function STEVE_ver28/Sorbent Bed/CO2 Desorption/q_star1 ==
  data: P input; q_star output; T input; kl output
function [q_star,kl] = fcn(P, T)


R = 8.314; % gas constant (Pa*m3)/(K*mol)
%T = 298; % K temperature
pp = P*0.001; %kPa, c_t -> (mol/m3)

a01=2.219; %mol/kg
a02=3.602; %mol/kg
b01=5.886*10^(-8); % 1/kPa
b02=4.436*10^(-8); % 1/kPa
E1R=5401; %K
E2R=4197; %K
b1=b01*exp(E1R/T); % 1/kPa
b2=b02*exp(E2R/T); % 1/kPa

q_star=a01*b1*pp/(1+b1*pp)+a02*b2*pp/(1+b2*pp); %mol/kg

k0=15;  %Originally 57(failed) then 5(worked). Default 15
roh=1054; %kg/m3
c0=P/(T*8.314); %mol/m3
c0_n0=c0/(q_star*roh);
kl=k0*c0_n0; %1/s


% Ko = 4.31e-4; % 1/bar Toth param
% deltaH = 29.380; % kJ/mol heat of adsorption
% R = 8.314; % gas constant
% T = 298; % K temperature
% qm = 5.09; % max q for CO2
% p = 1.429; % mol/kg Toth param
% 
% Keq = Ko*exp(deltaH/(R*T));
% pp = c_t.*R.*T;
% %p=0.27+c_t/T;
% q_star = ((qm.*Keq).*pp)./((1+(Keq.*pp).^p).^(1./p));

end

== matlab function STEVE_ver28/Sorbent Bed/CO2 Adsorption/Constants1 ==
  data: eps output; vs output; time input; resid_CO2 input; V input; DL output; vi output; c_init output; cFeed output; delta_eps output; q_init output; CO2 input; T input; P input
function [ eps, vs, DL, vi,  c_init, cFeed, delta_eps, q_init] = fcn(time, resid_CO2, V, CO2,T, P)
n=10;
%calculate void fraction
L=0.508; %Length of bed [m]
ID=(1-2*0.049)*0.0254; %Bed ID [m], 1-in OD SS304 smooth bore tubing w/ 0.049-in wall
Ab = pi/4*ID^2; %Bed cross-sectional area [m^2]
M = 110.5; %Adsorbent mass [g]
PD=0.003175; %Pellet Diameter [m]
PL=0.006858; %Pellet Length [m]
Sp=pi*PD*PL+2*(pi/4*PD^2); %Pellet Surface Area [m^2]
Vp=pi/4*PD^2*PL; %Pellet Volume [m^3]
rho_p=1054; %Pellet Density [kg/m^3], Son 2018, Son et al. 2019
rho_b=610; %bulk sorbent density [kg/m3], http://www.adsorbentcn.com/13x.htm 
eps=1-(M/1000)/(Ab*L)/rho_p; 

%calculate DL 
%Re=
DL=0.000899; %!!!! Check if this is correct   m2/s

%Calculate other
vs=V/(pi*(ID/2)^2); %m/s  V->m3/s, r->m
vi = vs/eps; %m/s
delta_eps=(1-eps)/eps;
if time<5 %Basically only use this for first cycle
    q_init=zeros(n,1); %mol/m3
else
    q_init=ones(n,1);
    q_init=q_init.*resid_CO2/(n-1);
    q_init(n,1)=0;
end
%CO2 = 0.003;                  % percent in air - can be in put from Simulink
% Air_mw = 28.9647;            % molar weight of air g/mol
%cFeed = CO2*1000/22.4;
c_init=zeros(n,1); %mol/m3
cFeed = P*CO2/(T*8.314);%mol/m3
c_init(1,1)=cFeed; %mol/m3

end

== matlab function STEVE_ver28/Sorbent Bed/CO2 Adsorption/q_star1 ==
  data: c_t input; q_star output; T input
function q_star = fcn(c_t, T)


R = 8.314; % gas constant (Pa*m3)/(K*mol)
%T = 298; % K temperature
pp = c_t.*R.*T*0.001; %kPa, c_t -> (mol/m3)

a01=2.219; %mol/kg
a02=3.602; %mol/kg
b01=5.886*10^(-8); % 1/kPa
b02=4.436*10^(-8); % 1/kPa
E1R=5401; %K
E2R=4197; %K
b1=b01*exp(E1R/T); % 1/kPa
b2=b02*exp(E2R/T); % 1/kPa

q_star=a01.*b1.*pp./(1+b1.*pp)+a02.*b2.*pp./(1+b2.*pp); %mol/kg


% Ko = 4.31e-4; % 1/bar Toth param
% deltaH = 29.380; % kJ/mol heat of adsorption
% R = 8.314; % gas constant
% T = 298; % K temperature
% qm = 5.09; % max q for CO2
% p = 1.429; % mol/kg Toth param
% 
% Keq = Ko*exp(deltaH/(R*T));
% pp = c_t.*R.*T;
% %p=0.27+c_t/T;
% q_star = ((qm.*Keq).*pp)./((1+(Keq.*pp).^p).^(1./p));

end

== matlab function STEVE_ver28/Sorbent Bed/CO2 Adsorption/spatial_calc1 ==
  data: L input; D2cDz2 output; DcDz output; c input; CO2 input; T input; P input; eps input; Vs input; DL input
function [D2cDz2, DcDz] = fcn(L,c, CO2, T, P, eps, Vs, DL)
n=10;
DcDz=zeros(n,1);
D2cDz2=zeros(n,1);
x=L/n;
z = 0:x:L;                % Spatial mesh generation
%n = 11;  
zhalf = zeros(n-1,1);
zhalf(1:n-1)=(z(1:n-1)+z(2:n))/2;

%CO2 = 0.003;                  % percent in air - can be in put from Simulink
Air_mw = 28.9647;            % molar weight of air g/mol
cFeed = P*CO2/(T*8.314); %mol/m3

DcDz(1,1)=-(Vs/(eps*DL))*(cFeed-c(1,1));  % !!   mol/m4
%DcDz(1,1)=0;
D2cDz2(1,1)=0;
D2cDz2(n,1)=0;
DcDz(n,1)=0;

% Calculate change in concentration from 2 to n-1 nodes in the bed 
for i=2:n-1
    DcDz(i) = (c(i)-c(i-1))/(z(i)-z(i-1)); %mol/m4
    D2cDz2(i) = (zhalf(i)*(c(i+1)-c(i))/(z(i+1)-z(i)) - zhalf(i-1)*(c(i)-c(i-1))/(z(i)-z(i-1))) / (zhalf(i)-zhalf(i-1));
%     D2cDz2(i) = (c(i+1)-2*c(i)+c(i))/(dz)^2;
end

% Calculate DcDz and D2cDz2 at z=L for boundary condition 
% aka last node


%DcDz(n) = (c(n)-c(n-1))/(z(n)-z(n-1));
%D2cDz2(n) = -1.0/(z(n)-zhalf(n-1))*(c(n)-c(n-1))/(z(n)-z(n-1));
%D2cDz2(n) = (zhalf(i)*(-c(i))/(-z(i)) - zhalf(i-1)*(c(i)-c(i-1))/(z(i)-z(i-1))) / (zhalf(i)-zhalf(i-1));

end

== matlab function STEVE_ver28/Sorbent Bed/Sorbent Bed Pressure Drop Model (Ergun Equation) ==
  data: y output; V input; sig input
function y = fcn(V, sig)
 
% Set constants for the Ergun equation

if sig==1
    y=0;
else

L=0.508; %Length of bed [m]
ID=(1-2*0.049)*0.0254; %Bed ID [m], 1-in OD SS304 smooth bore tubing w/ 0.049-in wall
Ab = pi/4*ID^2; %Bed cross-sectional area [m^2]
M = 110.5; %Adsorbent mass [g]
PD=0.003175; %Pellet Diameter [m]
PL=0.006858; %Pellet Length [m]
Sp=pi*PD*PL+2*(pi/4*PD^2); %Pellet Surface Area [m^2]
Vp=pi/4*PD^2*PL; %Pellet Volume [m^3]
rho_p=1054; %Pellet Density [kg/m^3], Son 2018, Son et al. 2019
rho_b=610; %bulk sorbent density [kg/m3], http://www.adsorbentcn.com/13x.htm 
e=1-(M/1000)/(Ab*L)/rho_p; %Void fraction; determined from pellet mass, internal volume and pellet density
mu=0.00001814; %Fluid dynamic viscosity [Pa*s], 7/7/2021 experiment
rho=1.068; %Fluid density [kg/m^3], 7/7/2021 experiment
 
% Pressure drop calculation using the modified Ergun equation for 
% sphericity and wall friction [7. D. Metha, M.C. Hawley, Wall effect 
% in packed columns, % Ind. Eng. Chem. Process Des. Dev. (1969) 8, 2, 
% 280–282.  
% https://doi.org/10.1021/i260030a021]
 
if V<0
    Dp=2*(3*Vp/(4*pi))^(1/3);  % equivalent spherical pellet diameter [m]
    Vs=abs(V)/Ab*101325/93350*(273.15+20.7)/298.15; % superficial velocity [m/s]
    phi_s=(6/Dp)/(Sp/Vp); % sphericity
    F = 1+4*Dp/(6*ID*(1-e)); % wall friction
    u=150*(1-e)^2/e^3*(mu*Vs*L)/(phi_s^2*Dp^2)*F^2+1.75*(1-e)/e^3*(rho*Vs^2*L)/(phi_s*Dp)*F;  %Modified Ergun eqn to calc DeltaP
    y=u; % Make it a negative value to subtract the calculated pressure from the inlet pressure  
else
    Dp=2*(3*Vp/(4*pi))^(1/3);  % equivalent spherical pellet diameter [m]
    Vs=V/Ab*101325/93350*(273.15+20.7)/298.15; % superficial velocity [m/s]
    phi_s=(6/Dp)/(Sp/Vp); % sphericity
    F = 1+4*Dp/(6*ID*(1-e)); % wall friction
    u=150*(1-e)^2/e^3*(mu*Vs*L)/(phi_s^2*Dp^2)*F^2+1.75*(1-e)/e^3*(rho*Vs^2*L)/(phi_s*Dp)*F;  %Modified Ergun eqn to calc DeltaP
    y=-u; % Make it a negative value to subtract the calculated pressure from the inlet pressure  
end

end
%Other parameter units
%V: Flow rate [m^3/s]



% % Set constants for Ergun eqution
% L=0.508; %Length of bed [m]
% e=0.67; %Void fraction 
% ID=0.02362; %Bed ID [m]
% Ab = pi/4*ID^2; %Bed cross-sectional area [m^2]
% PD=0.003175; %Pellet Diameter [m]
% PL=0.006858; %Pellet Length [m]
% Sp=pi*PD*PL; %Pellet Surface Area [m^2]
% Vp=pi/4*PD^2*PL; %Pellet Volume [m^3]
% mu=0.00001715; %Fluid dynamic viscosity [Pa*s]
% rho=1.292; %Fluid density [kg/m^3]
% 
% %Pressure drop calculation using the modified Ergun equation
% Dp=2*(3*Vp/(4*pi))^(1/3);  % equivalent spherical pellet diameter [m]
% Vs=V/Ab; % superficial velocity [m/s]
% phi_s=(6/Dp)/(Sp/Vp); %sphericity
% u=150*mu*(1-e)^2*Vs*L/(phi_s^2*e^3*Dp^2)+1.75*(1-e)*rho*Vs^2*L/(phi_s*e^3*Dp);  %Modified Ergun eqn to calc DeltaP
% 
% y=-u;

% if V>0
%     y=-u; % Make it a negative value to subtract the calculated pressure from the inlet pressure 
% elseif V==0
%     y=0;
% else
%     y=u;
% end
%Other parameter units
%V: Flow rate [m^3/s]

== matlab function STEVE_ver28/DAQ/MATLAB Function3 ==
  settings: updateMethod=DISCRETE  sampleTime=1
  data: UpO2 output; UpVol input; UpCO2 input
function UpO2  = fcn(UpVol,UpCO2)

UpVol=abs(UpVol);
UpCO2=abs(UpCO2);

if UpVol==0
UpO2=0;
else
VolCO2=UpVol*UpCO2;
VolO2=(UpVol-VolCO2)*0.21;
UpO2=(VolO2/UpVol)*100;

end

== matlab function STEVE_ver28/DAQ/MATLAB Function1 ==
  settings: updateMethod=DISCRETE  sampleTime=1
  data: CO2up output; x input; s input
function CO2up  = fcn(x,s)
if x<=0.003
sigma=0.00004;
else
sigma=x*0.02;
end
CO2=normrnd(x,sigma/3,[1,1000])*100;
CO2up=CO2(1,s);

== matlab function STEVE_ver28/DAQ/Cycle Counter ==
  data: t input; t_tot input; cycle output
function cycle  = fcn(t,t_tot)

cycle=floor(t/t_tot);  
  
  end

== matlab function STEVE_ver28/DAQ/MATLAB Function2 ==
  settings: updateMethod=DISCRETE  sampleTime=1
  data: CO2up output; x input; s input
function CO2up  = fcn(x,s)
if x<=0.003
sigma=0.00004;
else
sigma=x*0.02;
end
CO2=normrnd(x,sigma/3,[1,1000])*100;
CO2up=CO2(1,s);

== matlab function STEVE_ver28/DAQ/Upstream Flow Rate ==
  settings: updateMethod=DISCRETE  sampleTime=1
  data: FMup output; x input; s input
function FMup  = fcn(x,s)

range=10;
sigma=0.002*range+0.008*abs(x);
FM=normrnd(x,sigma/3,[1,1000]);
FMup=FM(1,s);

== matlab function STEVE_ver28/DAQ/RH to Dew Point ==
  settings: updateMethod=DISCRETE  sampleTime=1
  data: RH_Down input; DPT_Up output; DPT_Down output; RH_Up input; Temp_Down input; Temp_Up input
function [DPT_Up, DPT_Down]  = fcn(RH_Down, RH_Up, Temp_Down, Temp_Up)

b = 17.62;
c = 243.5;
gamma_up = log(RH_Up/100) + b*Temp_Up./(c+Temp_Up);
gamma_down = log(RH_Down/100) + b*Temp_Down./(c+Temp_Down);
DPT_Up = c*gamma_up./(b-gamma_up);
DPT_Down = c*gamma_down./(b-gamma_down);

end

== matlab function STEVE_ver28/DAQ/MATLAB Function4 ==
  settings: updateMethod=DISCRETE  sampleTime=1
  data: DnO2 output; DnVol input; DnCO2 input
function DnO2  = fcn(DnVol,DnCO2)

DnVol=abs(DnVol);
DnCO2=abs(DnCO2);

if DnVol==0
DnO2=0;
else
VolCO2=DnVol*DnCO2;
VolO2=(DnVol-VolCO2)*0.21;
DnO2=(VolO2/DnVol)*100;

end
